simulink model "Sim37"  (R2019a)
settings: Solver=FixedStepAuto  StartTime=0.0  StopTime=10.0  FixedStep=0.0001  RelTol=1e-3
settings Model: Creator=fbleo  LastModifiedBy=fbleo

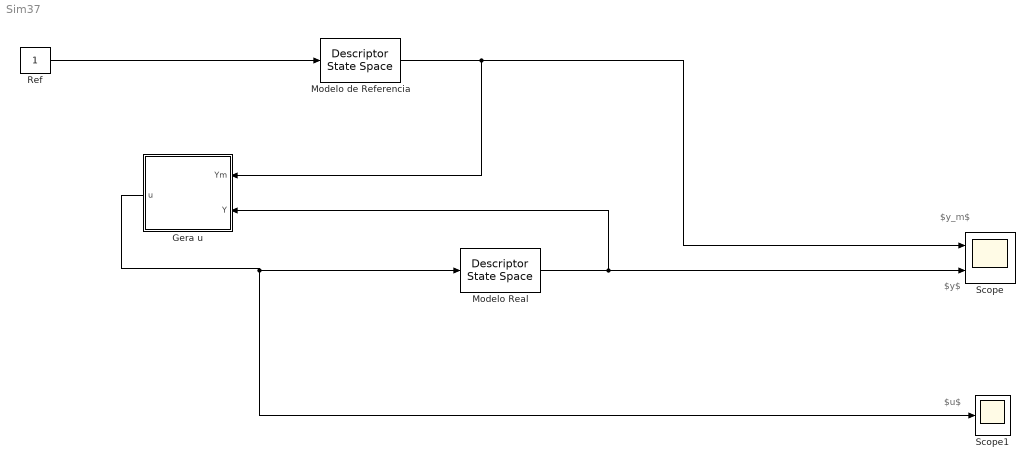
== system Sim37 ==
  note: $u$
  note: $y_m$
  note: $y$
  Gera u : Subsystem
  Modelo Real : DescriptorStateSpace  A=-1  B=2  D=0  InitialCondition=0.5
  Modelo de Referencia : DescriptorStateSpace  A=-3  B=3  D=0  InitialCondition=0
  Ref : Constant
  Scope : Scope  NumInputPorts=2
  Scope1 : Scope
  wires:
  Modelo de Referencia/1 -> Scope/1, Gera u/1(Ym)
  Gera u/1(u) -> Modelo Real/1, Scope1/1
  Ref/1 -> Modelo de Referencia/1
  Modelo Real/1 -> Scope/2, Gera u/2(Y)

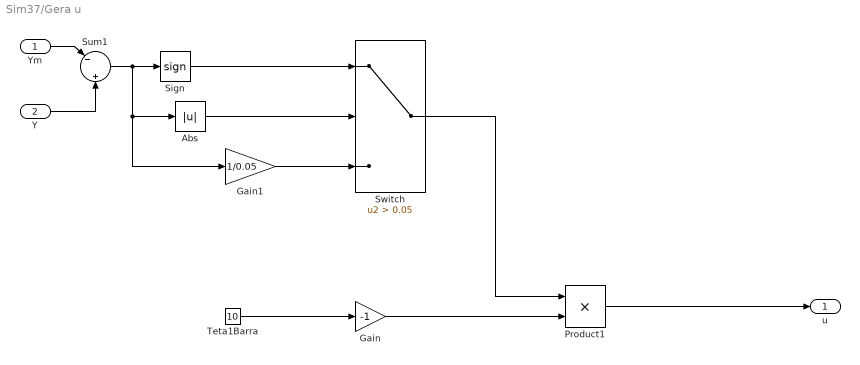
== system Sim37/Gera u ==
  Ym : Inport
  Y : Inport  Port=2
  Abs : Abs
  Gain : Gain  Gain=-1
  Gain1 : Gain  Gain=1/0.05
  Product1 : Product
  Sign : Signum
  Sum1 : Sum  Inputs=|-||+
  Switch : Switch  Criteria=u2 > Threshold  Threshold=0.05
  Teta1Barra : Constant  Value=10
  u : Outport
  wires:
  Ym/1 -> Sum1/1
  Y/1 -> Sum1/2
  Product1/1 -> u/1
  Gain/1 -> Product1/2
  Teta1Barra/1 -> Gain/1
  Switch/1 -> Product1/1
  Sign/1 -> Switch/1
  Sum1/1 -> Gain1/1, Abs/1, Sign/1
  Abs/1 -> Switch/2
  Gain1/1 -> Switch/3
